simulink model "my_model"  (R2019b)
settings: Solver=VariableStepAuto  StartTime=0.0  StopTime=10.0  RelTol=1e-3
settings Model: Creator=admin  LastModifiedBy=admin
settings DataIOCC: ReturnWorkspaceOutputs=off

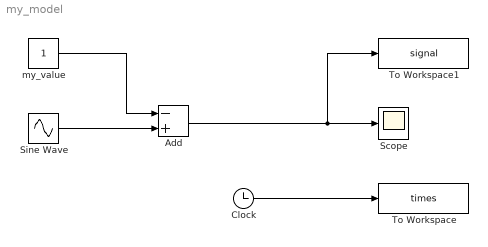
== system my_model ==
  Add : Sum  Inputs=-+
  Clock : Clock
  Scope : Scope
  Sine Wave : Sin  SampleTime=0
  To Workspace : ToWorkspace  VariableName=times  SampleTime=-1
  To Workspace1 : ToWorkspace  VariableName=signal  SampleTime=-1
  my_value : Constant
  wires:
  Sine Wave/1 -> Add/2
  Add/1 -> To Workspace1/1, Scope/1
  my_value/1 -> Add/1
  Clock/1 -> To Workspace/1
